simulink model "Single_Degree_of_Freedom"  (R2023b)
settings: configuration reference "ClusterControlConfig" (kept outside this file)
undefined symbols (not defined in the file or in its folder): DiscIntNeverNeededParam
libraries: simulink x1
settings Model: DataDictionary=ClusterControl.sldd  Creator=joels  LastModifiedBy=joel
settings ConfigSetRef: SourceName=ClusterControlConfig

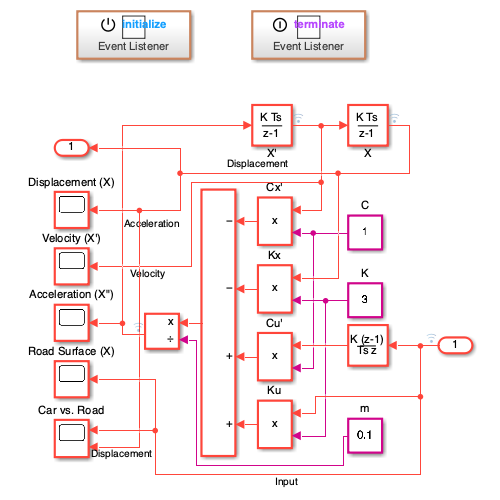
[thumbnail: Simulink's stored preview of the top-level diagram]
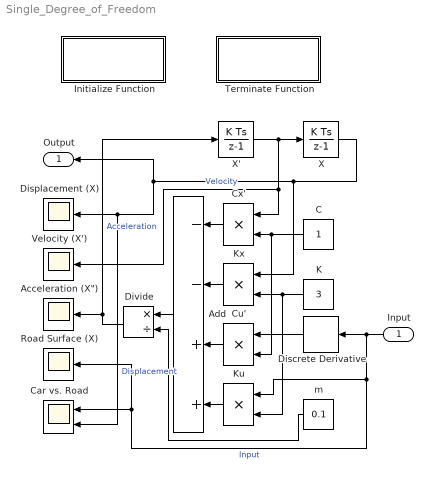
== system Single_Degree_of_Freedom ==
  Input : Inport
  "Acceleration (X\")" : Scope
  Add : Sum  Inputs=--++
  C : Constant
  Car vs. Road : Scope  NumInputPorts=2
  Cu' : Product
  Cx' : Product
  Discrete Derivative : simulink/Discrete/Discrete Derivative  gainval=1.0  ICPrevScaledInput=0.0  OutMin=[]  OutMax=[]  OutDataType=fixdt(1, 16)  OutScaling=2^-10  DoSatur=off
  Displacement (X) : Scope
  Divide : Product  Inputs=*/
  Initialize Function : Subsystem  TreatAsAtomicUnit=on
  K : Constant  Value=3
  Ku : Product
  Kx : Product
  Road Surface (X) : Scope
  Terminate Function : Subsystem  TreatAsAtomicUnit=on
  Velocity (X') : Scope
  X : DiscreteIntegrator  SampleTime=-1  ICPrevOutput=DiscIntNeverNeededParam  ICPrevScaledInput=DiscIntNeverNeededParam
  X' : DiscreteIntegrator  SampleTime=-1  ICPrevOutput=DiscIntNeverNeededParam  ICPrevScaledInput=DiscIntNeverNeededParam
  m : Constant  Value=0.1
  Output : Outport
  wires:
  Discrete Derivative/1 -> Cu'/1
  Kx/1 -> Add/2
  Cu'/1 -> Add/3
  Ku/1 -> Add/4
  m/1 -> Divide/2
  Add/1 -> Divide/1
  Divide/1 -> X'/1, "Acceleration (X\")"/1  "Acceleration"
  Cx'/1 -> Add/1
  C/1 -> Cu'/2, Cx'/2
  Input/1 -> Discrete Derivative/1, Ku/1, Car vs. Road/1, Road Surface (X)/1  "Input"
  X'/1 -> X/1, Velocity (X')/1, Cx'/1  "Velocity"
  X/1 -> Output/1, Car vs. Road/2, Displacement (X)/1, Kx/1  "Displacement"
  K/1 -> Ku/2, Kx/2

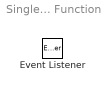
== system Single_Degree_of_Freedom/Initialize Function ==
  Event Listener : EventListener  DisableCoverage=on  EventName=reset

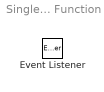
== system Single_Degree_of_Freedom/Terminate Function ==
  Event Listener : EventListener  DisableCoverage=on  EventType=Terminate  EventName=reset
